simulink model "Lab1_2"  (R2024b)
settings: Solver=FixedStepAuto  StartTime=0.0  StopTime=inf  FixedStep=0.01  RelTol=1e-3  EnableMultiTasking=on
libraries: stm32f4xxblockslib x4, stm32g4xxblockslib x3
settings Model: STM32="{\"EncoderBlockForG4\":[{\"ID\":\"untitled1:1\"},{\"ID\":\"qei:3\"},{\"ID\":\"qei:40\"},{\"ID\":\"qei:46\"}],\"DigitalPortRead\":[{\"ID\":\"qei:12\"},{\"ID\":\"qei:17\"},{\"ID\":\"qei:48\"},{\"ID\":\"qei:52\"}]}"  SimulationMode=external  Creator=ACER  LastModifiedBy=ACER
settings OptimizationCC: DefaultParameterBehavior=Inlined  EnhancedBackFolding=on  PassReuseOutputArgsAs=Individual arguments  ZeroExternalMemoryAtStartup=off  ZeroInternalMemoryAtStartup=off  MaxStackSize=512  OptimizeBlockOrder=speed  DifferentSizesBufferReuse=on  OptimizationCustomize=off  EfficientTunableParamExpr=on
settings DebuggingCC: ParameterTunabilityLossMsg=error
settings HardwareCC: ProdBitPerPointer=32  ProdBitPerSizeT=32  ProdBitPerPtrDiffT=32  ProdLargestAtomicInteger=Long  ProdLargestAtomicFloat=Double  ProdWordSize=32  ProdLongLongMode=on  ProdHWDeviceType=ARM Compatible->ARM Cortex-M
settings SFSimCC: MATLABDynamicMemAlloc=off
settings RTWCC: Description=Embedded Coder  SystemTargetFile=ert.tlc  HardwareBoard=STM32G4xx Based  TemplateMakefile=ert_default_tmf  Toolchain=GNU Tools for ARM Embedded Processors
settings CodeAppCC: ForceParamTrailComments=on  IgnoreCustomStorageClasses=off  OperatorAnnotations=on  SimulinkDataObjDesc=on  SFDataObjDesc=on  InsertBlockDesc=on
settings ERTTargetCC: TargetLangStandard=C99 (ISO)  CodeReplacementLibrary=ARM Cortex-M  ExtModeTransport=3  ExtModeStaticAlloc=on  ExtModeStaticAllocSize=2048  ExtModeMexFile=ext_xcp  ExtModeIntrfLevel=Level2 - Open

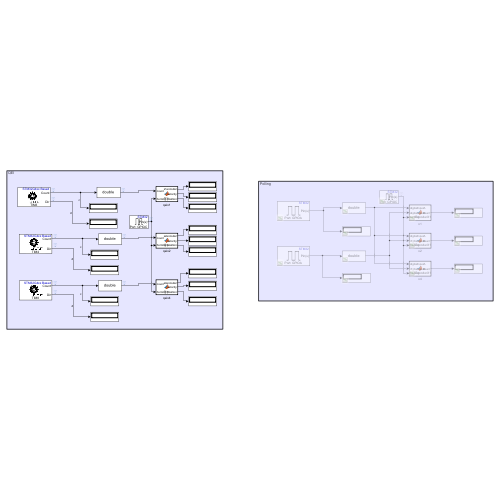
[thumbnail: Simulink's stored preview of the top-level diagram]
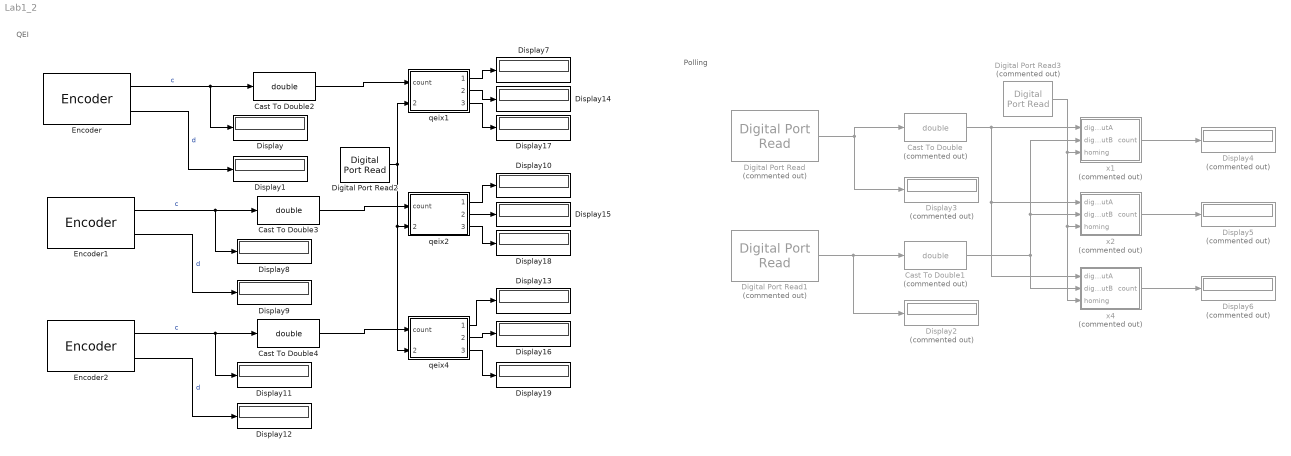
== system Lab1_2 ==
  note: QEI
  note: Polling
  Cast To Double : DataTypeConversion  Commented=on  OutDataTypeStr=double  SaturateOnIntegerOverflow=off  RndMeth=Floor
  Cast To Double1 : DataTypeConversion  Commented=on  OutDataTypeStr=double  SaturateOnIntegerOverflow=off  RndMeth=Floor
  Cast To Double2 : DataTypeConversion  OutDataTypeStr=double  SaturateOnIntegerOverflow=off  RndMeth=Floor
  Cast To Double3 : DataTypeConversion  OutDataTypeStr=double  SaturateOnIntegerOverflow=off  RndMeth=Floor
  Cast To Double4 : DataTypeConversion  OutDataTypeStr=double  SaturateOnIntegerOverflow=off  RndMeth=Floor
  Digital Port Read : stm32f4xxblockslib/Digital Port Read  Commented=on  PortName=GPIOA  PinNumber=6  ReadOperation=on  IOAsArray=on  SampleTime=-1  EnableSimPort=off  hoistedMaskSrc=ECSoC/ECSimCodegen/Digital Port Read
      settings: LibrarySourceBlock=stm32g4xxblockslib/Digital Port Read
  Digital Port Read1 : stm32f4xxblockslib/Digital Port Read  Commented=on  PortName=GPIOA  PinNumber=7  ReadOperation=on  IOAsArray=on  SampleTime=-1  EnableSimPort=off  hoistedMaskSrc=ECSoC/ECSimCodegen/Digital Port Read
      settings: LibrarySourceBlock=stm32g4xxblockslib/Digital Port Read
  Digital Port Read2 : stm32f4xxblockslib/Digital Port Read  PortName=GPIOC  PinNumber=13  ReadOperation=on  IOAsArray=on  SampleTime=-1  EnableSimPort=off  hoistedMaskSrc=ECSoC/ECSimCodegen/Digital Port Read
      settings: LibrarySourceBlock=stm32g4xxblockslib/Digital Port Read
  Digital Port Read3 : stm32f4xxblockslib/Digital Port Read  Commented=on  PortName=GPIOC  PinNumber=13  ReadOperation=on  IOAsArray=on  SampleTime=-1  EnableSimPort=off  hoistedMaskSrc=ECSoC/ECSimCodegen/Digital Port Read
      settings: LibrarySourceBlock=stm32g4xxblockslib/Digital Port Read
  Display{,1,7..19} (15 alike) : Display
  Display{2..6} (5 alike) : Display  Commented=on
  Encoder : stm32g4xxblockslib/Encoder  TimerModule=TIM3  EnableResetInput=off  OutputCountAfterFirstIndex=off  OutputValidIndex=off  OutputDirection=on  OutputStatus=off  SampleTime=-1
  Encoder1 : stm32g4xxblockslib/Encoder  TimerModule=TIM4  EnableResetInput=off  OutputCountAfterFirstIndex=off  OutputValidIndex=off  OutputDirection=on  OutputStatus=off  SampleTime=-1
  Encoder2 : stm32g4xxblockslib/Encoder  TimerModule=TIM8  EnableResetInput=off  OutputCountAfterFirstIndex=off  OutputValidIndex=off  OutputDirection=on  OutputStatus=off  SampleTime=-1
  qeix1 : MATLAB Function  TreatAsAtomicUnit=on
  qeix2 : MATLAB Function  TreatAsAtomicUnit=on
  qeix4 : MATLAB Function  TreatAsAtomicUnit=on
  x1 : MATLAB Function  Commented=on  TreatAsAtomicUnit=on
  x2 : MATLAB Function  Commented=on  TreatAsAtomicUnit=on
  x4 : MATLAB Function  Commented=on  TreatAsAtomicUnit=on
  wires:
  Encoder/1 -> Cast To Double2/1, Display/1  "c"
  Encoder/2 -> Display1/1  "d"
  Digital Port Read/1 -> Display3/1, Cast To Double/1
  Digital Port Read1/1 -> Display2/1, Cast To Double1/1
  Cast To Double/1 -> x4/1(digitalInputA), x2/1(digitalInputA), x1/1(digitalInputA)
  x1/1(count) -> Display4/1
  Cast To Double1/1 -> x2/2(digitalInputB), x1/2(digitalInputB), x4/2(digitalInputB)
  x2/1(count) -> Display5/1
  x4/1(count) -> Display6/1
  qeix1/1(x1encoder) -> Display7/1
  Cast To Double2/1 -> qeix1/1(count)
  Cast To Double3/1 -> qeix2/1(count)
  qeix2/1(x2encoder) -> Display10/1
  Encoder1/1 -> Cast To Double3/1, Display8/1  "c"
  Encoder1/2 -> Display9/1  "d"
  Cast To Double4/1 -> qeix4/1(count)
  qeix4/1(x4encoder) -> Display13/1
  Encoder2/1 -> Cast To Double4/1, Display11/1  "c"
  Encoder2/2 -> Display12/1  "d"
  Digital Port Read2/1 -> qeix1/2(homing), qeix4/2(homing), qeix2/2(homing)
  qeix1/2(velocity) -> Display14/1
  qeix2/2(velocity) -> Display15/1
  qeix4/2(velocity) -> Display16/1
  Digital Port Read3/1 -> x4/3(homing), x2/3(homing), x1/3(homing)
  qeix1/3(position) -> Display17/1
  qeix2/3(position) -> Display18/1
  qeix4/3(position) -> Display19/1

== matlab function Lab1_2/x2 ==
  data: digitalInputA input; count output; digitalInputB input; homing input
function count = readEncoderX1(digitalInputA, digitalInputB,homing)
    persistent encoderCount;

    if isempty(encoderCount)
        encoderCount = 0;
    end

    persistent lastA;
    if isempty(lastA)
        lastA = digitalInputA;
    end
    if homing > 0
        encoderCount = 0;
        lastA = digitalInputA;
    end
    if lastA ~= digitalInputA
        if digitalInputA == 0 &&  digitalInputB == 1 && lastA == 1
            encoderCount = encoderCount + 1;
        elseif digitalInputA == 0 &&  digitalInputB == 0 && lastA == 1
            encoderCount = encoderCount - 1;
        elseif digitalInputA == 1 &&  digitalInputB == 0 && lastA == 0 
            encoderCount = encoderCount + 1;
        elseif digitalInputA == 1 &&  digitalInputB == 1 && lastA == 0
            encoderCount = encoderCount - 1;
        end
        lastA = digitalInputA;
    end 
    % กำหนดค่าที่จะ return
    count = encoderCount;
end

== matlab function Lab1_2/x1 ==
  data: digitalInputA input; digitalInputB input; count output; homing input
function count = readEncoderX1(digitalInputA, digitalInputB, homing)
    persistent encoderCount;

    if isempty(encoderCount)
        encoderCount = 0;
    end

    persistent lastA;
    if isempty(lastA)
        lastA = digitalInputA;
    end
    if homing > 0
        encoderCount = 0;
        lastA = digitalInputA;
    end
    if lastA ~= digitalInputA
        if digitalInputA == 0 &&  digitalInputB == 1 && lastA == 1
            encoderCount = encoderCount + 1;
        elseif digitalInputA == 0 &&  digitalInputB == 0 && lastA == 1
            encoderCount = encoderCount - 1;
        end
        lastA = digitalInputA;
    end 
    count = encoderCount;
end

== matlab function Lab1_2/x4 ==
  data: digitalInputA input; count output; digitalInputB input; homing input
function count = readEncoderX1(digitalInputA, digitalInputB,homing)
    persistent encoderCount;

    if isempty(encoderCount)
        encoderCount = 0;
    end

    persistent lastA;
    if isempty(lastA)
        lastA = digitalInputA;
    end
    persistent lastB;
    if isempty(lastB)
        lastB = digitalInputB;
    end
    if homing > 0
        encoderCount = 0;
        lastA = digitalInputA;
        lastB = digitalInputB;
    end
    if digitalInputA == 0 &&  digitalInputB == 1 && lastA == 1
        encoderCount = encoderCount + 1;
    elseif digitalInputA == 0 &&  digitalInputB == 0 && lastA == 1
        encoderCount = encoderCount - 1;
    elseif digitalInputA == 1 &&  digitalInputB == 0 && lastA == 0 
        encoderCount = encoderCount + 1;
    elseif digitalInputA == 1 &&  digitalInputB == 1 && lastA == 0
        encoderCount = encoderCount - 1;
    elseif digitalInputB == 0 &&  digitalInputA == 0 && lastB == 1
        encoderCount = encoderCount + 1;
    elseif digitalInputB == 0 &&  digitalInputA == 1 && lastB == 1
        encoderCount = encoderCount - 1;
    elseif digitalInputB == 1 &&  digitalInputA == 1 && lastB == 0 
        encoderCount = encoderCount + 1;
    elseif digitalInputB == 1 &&  digitalInputA == 0 && lastB == 0
        encoderCount = encoderCount - 1;
    end
    lastA = digitalInputA;
    lastB = digitalInputB;
    % กำหนดค่าที่จะ return
    count = encoderCount;
end

== matlab function Lab1_2/qeix1 ==
  data: count input; x1encoder output; homing input; velocity output; position output
function [x1encoder, velocity,position] = fcn(count, homing)
    persistent encoderCount;
    persistent prev_Count;
    persistent prev_EncoderCount;
    
    PPR = 24;  
    
    if isempty(prev_Count)
        prev_Count = count;
    end
    if isempty(encoderCount)
        encoderCount = 0;
    end
    if isempty(prev_EncoderCount)
        prev_EncoderCount = 0;
    end
    
    if homing > 0
        prev_Count = count;
        encoderCount = 0;
        prev_EncoderCount = 0;
    end
    if prev_Count > 65000 && count < 1000
        encoderCount = encoderCount + (count + (65520 - prev_Count));
    elseif prev_Count < 1000 && count > 65000
        encoderCount = encoderCount - ((65520 - count) + prev_Count);
    else
        encoderCount = encoderCount + (count - prev_Count);
    end

    deltaCount = encoderCount - prev_EncoderCount;
    velocity = (deltaCount / PPR);  
    position = (encoderCount/ PPR) *2 ;
    samplingRate = 100;  
    velocity = velocity * samplingRate * 2 * pi;
    prev_Count = count;
    prev_EncoderCount = encoderCount;
    x1encoder = encoderCount;
end

== matlab function Lab1_2/qeix2 ==
  data: count input; x2encoder output; homing input; velocity output; position output
function [x2encoder, velocity,position] = fcn(count, homing)
    persistent encoderCount;
    persistent prev_Count;
    persistent prev_EncoderCount;
    
    
    PPR = 24;  
    
    if isempty(prev_Count)
        prev_Count = count;
    end
    if isempty(encoderCount)
        encoderCount = 0;
    end
    if isempty(prev_EncoderCount)
        prev_EncoderCount = 0;
    end
    
    if homing > 0
        prev_Count = count;
        prev_EncoderCount = 0;
        encoderCount = 0;
    end
    if prev_Count > 65000 && count < 1000
        encoderCount = encoderCount + (count + (65520 - prev_Count));
    elseif prev_Count < 1000 && count > 65000
        encoderCount = encoderCount - ((65520 - count) + prev_Count);
    else
        encoderCount = encoderCount + (count - prev_Count);
    end

    deltaCount = encoderCount - prev_EncoderCount;
    velocity = (deltaCount / PPR); 
    position = (encoderCount/ PPR);

    samplingRate = 100;  
    velocity =  velocity * samplingRate *2* pi;
    prev_Count = count;
    prev_EncoderCount = encoderCount;

    % Return encoder count
    x2encoder = encoderCount;
end

== matlab function Lab1_2/qeix4 ==
  data: count input; x4encoder output; homing input; velocity output; position output
function [x4encoder, velocity,position] = fcn(count, homing)
    persistent encoderCount;
    persistent prev_Count;
    persistent prev_EncoderCount;
    
    % จำนวนพัลส์ต่อรอบ (PPR)
    PPR = 24;  % กำหนดค่า PPR ของ Encoder ตามที่ใช้งาน
    
    if isempty(prev_Count)
        prev_Count = count;
    end
    if isempty(encoderCount)
        encoderCount = 0;
    end
    if isempty(prev_EncoderCount)
        prev_EncoderCount = 0;
    end
    
    if homing > 0
        prev_Count = count;
        prev_EncoderCount = 0;
        encoderCount = 0;
    end
    if prev_Count > 65000 && count < 1000
        encoderCount = encoderCount + (count + (65520 - prev_Count));
    elseif prev_Count < 1000 && count > 65000
        encoderCount = encoderCount - ((65520 - count) + prev_Count);
    else
        encoderCount = encoderCount + (count - prev_Count);
    end

    deltaCount = encoderCount - prev_EncoderCount;
    velocity = (deltaCount / PPR); 
    position = (encoderCount/ PPR)/2;

    samplingRate = 100;  
    velocity = velocity * samplingRate *2* pi; 

    % Update previous counts
    prev_Count = count;
    prev_EncoderCount = encoderCount;

    % Return encoder count
    x4encoder = encoderCount;
end
